simulink model "d_q_transform_and_pll"  (R2019a)
settings: Solver=VariableStepAuto  StartTime=0.0  StopTime=2  MaxStep=1e-4  RelTol=1e-4
values from neighbouring files (symbols this model uses):
  Kipll = Kpll/Tpll    [d_q_trans_pll_script.m]
  Kpll = (1/Vm)*(1/(alfa*Ts))    [d_q_trans_pll_script.m]
  Vm = 230*sqrt(2)    [d_q_trans_pll_script.m]
libraries: simulink x1
settings Model: Creator=gsahi  LastModifiedBy=Görkem

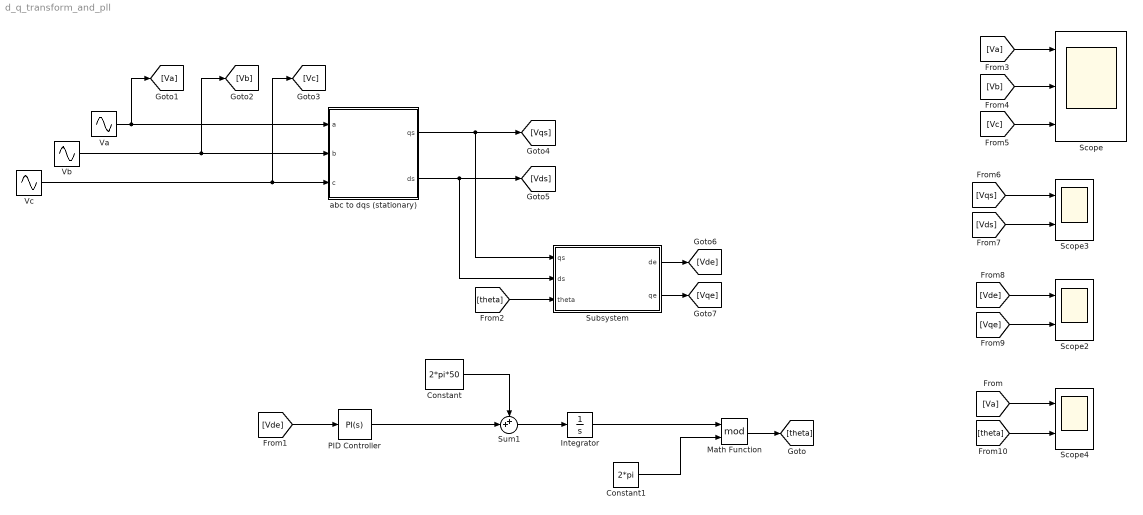
== system d_q_transform_and_pll ==
  Constant : Constant  Value=2*pi*50
  Constant1 : Constant  Value=2*pi
  Integrator : Integrator
  Math Function : Math  Operator=mod  SaturateOnIntegerOverflow=on
  PID Controller : simulink/Continuous/PID Controller  Controller=PI  Form=Parallel  TimeDomain=Continuous-time  SampleTime=-1  IntegratorMethod=Forward Euler  FilterMethod=Forward Euler  ControllerParametersSource=internal  P=Kpll  I=Kipll  D=0  UseFilter=on  N=100  TunerSelectOption=Transfer Function Based (PID Tuner App)  InitialConditionSource=internal  InitialConditionForIntegrator=0  InitialConditionForFilter=0  DifferentiatorICPrevScaledInput=0  ExternalReset=none  TrackingMode=off  Kt=1  LimitOutput=off  UpperSaturationLimit=inf  LowerSaturationLimit=-inf  LinearizeAsGain=on  AntiWindupMode=none  Kb=1  POutMin=[]  POutMax=[]  IOutMin=[]  IOutMax=[]  DOutMin=[]  DOutMax=[]  NOutMin=[]  NOutMax=[]  SumOutMin=[]  SumOutMax=[]  SaturationOutMin=[]  SaturationOutMax=[]  PParamMin=[]  PParamMax=[]  IParamMin=[]  IParamMax=[]  DParamMin=[]  DParamMax=[]  NParamMin=[]  NParamMax=[]  KbParamMin=[]  KbParamMax=[]  KtParamMin=[]  KtParamMax=[]  KbOutMin=[]  KbOutMax=[]  KtOutMin=[]  KtOutMax=[]  IntegratorOutMin=[]  IntegratorOutMax=[]  FilterOutMin=[]  FilterOutMax=[]  SumI1OutMin=[]  SumI1OutMax=[]  SumI2OutMin=[]  SumI2OutMax=[]  SumI3OutMin=[]  SumI3OutMax=[]  SumI4OutMin=[]  SumI4OutMax=[]  SumDOutMin=[]  SumDOutMax=[]  DifferentiatorOutMin=[]  DifferentiatorOutMax=[]  FilterDiffOutCoefMin=[]  FilterDiffOutCoefMax=[]  ReciprocalOutMin=[]  ReciprocalOutMax=[]  SumDenOutMin=[]  SumDenOutMax=[]  SumNumOutMin=[]  SumNumOutMax=[]  DivideOutMin=[]  DivideOutMax=[]  IntegratorContinuousStateAttributes=''  IntegratorStateMustResolveToSignalObject=off  IntegratorRTWStateStorageClass=Auto  FilterContinuousStateAttributes=''  FilterStateMustResolveToSignalObject=off  FilterRTWStateStorageClass=Auto  ParallelPVariant=InternalParameters  IdealPVariant=Disabled  IVariant=InternalParameters  DVariant=Disabled  IntegratorVariant=Continuous  SatVariant=Disabled  AWVariant=Passthrough  PCopyVariant=Disabled  TRVariant=Disabled  FdbkBlocksVariant=Forward  IdealPFdbkVariant=Disabled  SatFdbkVariant=Disabled  DerivativeFilterVariant=Disabled  NVariant=Disabled  NCopyVariant=Disabled_SignalSpec  FilterICVariant=Disabled  IntegratorICVariant=InternalICs  ExternalResetVariant=Disabled  TRSumVariant=Passthrough  SumFdbkVariant=Disabled  SumVariant=Sum_PI
  Scope : Scope  NumInputPorts=3
  Scope2 : Scope  NumInputPorts=2
  Scope3 : Scope  NumInputPorts=2
  Scope4 : Scope  NumInputPorts=2
  Subsystem : Subsystem
  Sum1 : Sum  Inputs=++|
  Va : Sin  Amplitude=Vm  Frequency=2*pi*50  SampleTime=0
  Vb : Sin  Amplitude=Vm  Frequency=2*pi*50  Phase=-2*pi/3  SampleTime=0
  Vc : Sin  Amplitude=Vm  Frequency=2*pi*50  Phase=-4*pi/3  SampleTime=0
  abc to dqs (stationary) : Subsystem
  wires:
  Va/1 -> abc to dqs (stationary)/1(a), [Va]
  Vb/1 -> abc to dqs (stationary)/2(b), [Vb]
  Vc/1 -> abc to dqs (stationary)/3(c), [Vc]
  abc to dqs (stationary)/1(qs) -> Subsystem/1("qs "), [Vqs]
  abc to dqs (stationary)/2(ds) -> Subsystem/2("ds "), [Vds]
  Integrator/1 -> Math Function/1
  PID Controller/1 -> Sum1/2
  Sum1/1 -> Integrator/1
  Math Function/1 -> [theta]
  Constant1/1 -> Math Function/2
  Constant/1 -> Sum1/1
  Subsystem/1("de ") -> [Vde]
  [Vde] -> PID Controller/1
  Subsystem/2("qe ") -> [Vqe]
  [theta] -> Subsystem/3(theta)
  [Va] -> Scope/1
  [Vb] -> Scope/2
  [Vc] -> Scope/3
  [Vqs] -> Scope3/1
  [Vds] -> Scope3/2
  [Vqe] -> Scope2/2
  [Vde] -> Scope2/1
  [Va] -> Scope4/1
  [theta] -> Scope4/2

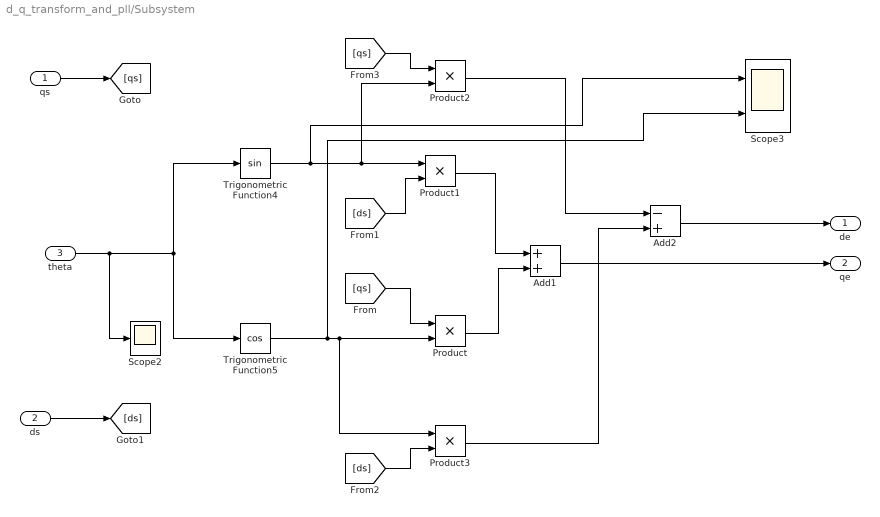
== system d_q_transform_and_pll/Subsystem ==
  "qs " : Inport
  "ds " : Inport  Port=2
  theta : Inport  Port=3
  Add1 : Sum
  Add2 : Sum  Inputs=-+
  Product{,1..3} (4 alike) : Product
  Scope2 : Scope
  Scope3 : Scope  NumInputPorts=2
  Trigonometric Function4 : Trigonometry
  Trigonometric Function5 : Trigonometry  Operator=cos
  "de " : Outport
  "qe " : Outport  Port=2
  wires:
  [ds] -> Product3/2
  theta/1 -> Scope2/1, Trigonometric Function4/1, Trigonometric Function5/1
  "ds "/1 -> [ds]
  Add2/1 -> "de "/1
  Product2/1 -> Add2/1
  [qs] -> Product/1
  "qs "/1 -> [qs]
  Product3/1 -> Add2/2
  [qs] -> Product2/1
  Add1/1 -> "qe "/1
  [ds] -> Product1/2
  Product/1 -> Add1/2
  Product1/1 -> Add1/1
  Trigonometric Function4/1 -> Product2/2, Product1/1, Scope3/1
  Trigonometric Function5/1 -> Product/2, Product3/1, Scope3/2

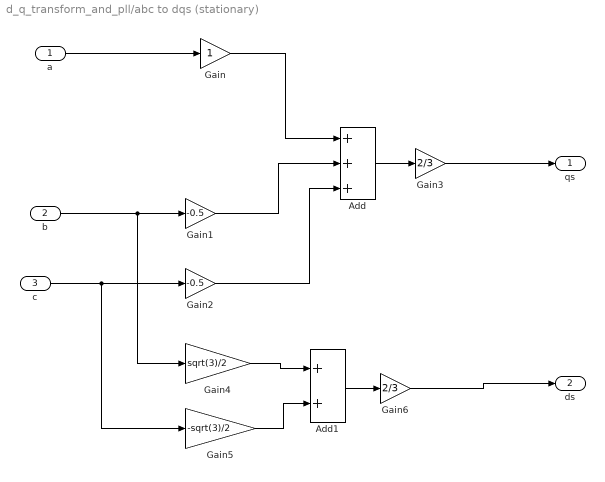
== system d_q_transform_and_pll/abc to dqs (stationary) ==
  a : Inport
  b : Inport  Port=2
  c : Inport  Port=3
  Add : Sum  Inputs=+++
  Add1 : Sum
  Gain : Gain
  Gain1 : Gain  Gain=-0.5
  Gain2 : Gain  Gain=-0.5
  Gain3 : Gain  Gain=2/3
  Gain4 : Gain  Gain=sqrt(3)/2
  Gain5 : Gain  Gain=-sqrt(3)/2
  Gain6 : Gain  Gain=2/3
  qs : Outport
  ds : Outport  Port=2
  wires:
  a/1 -> Gain/1
  Gain/1 -> Add/1
  Gain5/1 -> Add1/2
  Gain1/1 -> Add/2
  b/1 -> Gain4/1, Gain1/1
  c/1 -> Gain5/1, Gain2/1
  Add/1 -> Gain3/1
  Gain2/1 -> Add/3
  Gain4/1 -> Add1/1
  Gain3/1 -> qs/1
  Add1/1 -> Gain6/1
  Gain6/1 -> ds/1
